simulink model "TP09_Ej11"  (R2020b)
settings: Solver=FixedStepAuto  StartTime=0.0  StopTime=20e-3  FixedStep=1e-6  RelTol=1e-3  EnableMultiTasking=on
settings Model: Creator=54115  LastModifiedBy=Juan
settings DataIOCC: ReturnWorkspaceOutputs=off
settings OptimizationCC: LifeSpan=inf
settings DebuggingCC: SFUnexpectedBacktrackingDiag=warning  SFNoUnconditionalDefaultTransitionDiag=warning  ArithmeticOperatorsInVariantConditions=warning
settings SFSimCC: SimUseLocalCustomCode=off  CustomCodeUndefinedFunction=UseInterfaceOnly
settings RTWCC: RTWUseLocalCustomCode=off
settings CodeAppCC: StateflowObjectComments=on
settings GRTTargetCC: TargetLangStandard=C89/C90 (ANSI)
settings ConfigComp: CovMetricSettings=dw  CovSaveCumulativeToWorkspaceVar=on  CovSaveSingleToWorkspaceVar=on  CovExternalEMLEnable=off

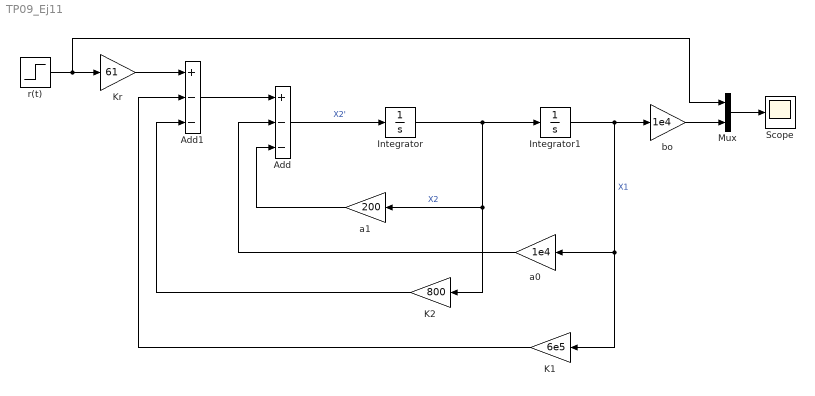
== system TP09_Ej11 ==
  Add : Sum  Inputs=+--
  Add1 : Sum  Inputs=+--
  Integrator : Integrator
  Integrator1 : Integrator
  K1 : Gain  Gain=6e5
  K2 : Gain  Gain=800
  Kr : Gain  Gain=61
  Mux : Mux  Inputs=2
  Scope : Scope
  a0 : Gain  Gain=1e4
  a1 : Gain  Gain=200
  bo : Gain  Gain=1e4
  r(t) : Step  Time=0  SampleTime=0
  wires:
  Integrator/1 -> Integrator1/1, K2/1, a1/1  "X2"
  a1/1 -> Add/3
  Integrator1/1 -> bo/1, K1/1, a0/1  "X1"
  Mux/1 -> Scope/1
  Add1/1 -> Add/1
  r(t)/1 -> Mux/1, Kr/1
  K2/1 -> Add1/3
  a0/1 -> Add/2
  K1/1 -> Add1/2
  bo/1 -> Mux/2
  Kr/1 -> Add1/1
  Add/1 -> Integrator/1  "X2'"
